simulink model "slcp"  (Simulink 6.3)
settings: Solver=ode5  SolverMode=SingleTasking  StartTime=0.0  StopTime=1000  FixedStep=.01  MaxStep=0.1  RelTol=1e-3  AbsTol=1e-6
PreLoadFcn:
  | initcp
undefined symbols (not defined in the file or in its folder): init_cond
libraries: fuzblock x1
CloseFcn:
  | AnimFigTitle = [winName, ': Cart & Pole Animation']; AnimFigH = findobj(0,'Name',AnimFigTitle); close(AnimFigH)
settings Model: Creator=pascal  LastModifiedBy=mhaselti  StrictBusMsg=None
settings DataIOCC: LimitDataPoints=off  SaveOutput=off  SaveTime=off
settings OptimizationCC: BlockReduction=off  BooleanDataType=off
settings DebuggingCC: SigSpecEnsureSampleTime=on  SolverPrmCheckMsg=none
settings HardwareCC: TargetUnknown=on
settings RTWCC: TemplateMakefile=grt_unix.tmf

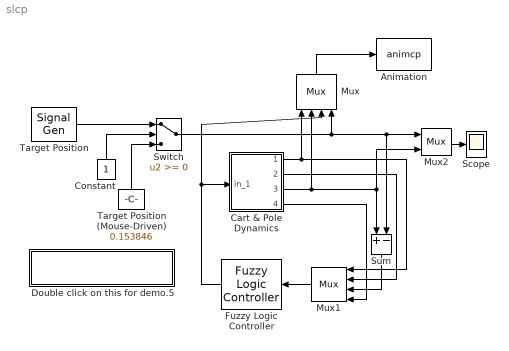
== system slcp ==
  Animation : S-Function  FunctionName=animcp
  Cart & Pole Dynamics : Subsystem  mask(Cart & Pole){init_cond =[0, 0, 0, 0],  specs =[1.0, 0.1, 1.0, 9.8]}
      mask prompts: init_cond  "Initial Conditions (angle, angular velocity, cart position and cart velocity):";  specs  "Physical Specifications (pole length, pole mass, cart mass and g):"
      mask help: Inverted Pendulum (cart & pole)
      mask init:
      | l=specs(1)/2;m=specs(2);mc=specs(3);g=specs(4);
      mask Help: Inverted Pendulum
      mask Display: plot(-4,-1,4,6,[0 3 2.8 -0.2 0],[1 5 5.15 1.15 1],[-1 -1 1 1 -1],[1 0 0 1 1],[-3.5 3.5],[0 0])
  Constant : Constant  Orientation=up
  Double click on this for demo.5 : Subsystem
      settings: OpenFcn=initcp
      mask Display: disp('Variable Initialization')
  Fuzzy Logic Controller : fuzblock/Fuzzy Logic  Controller  Orientation=left  fis=fismatrix
  Mux : Mux  Orientation=up
  Mux1 : Mux  Orientation=left
  Mux2 : Mux  Inputs=2
  Scope : Scope
      settings: TickLabels=on  TimeRange=10.000000  YMin=-2  YMax=2  DataFormat=Array
  Sum : Sum  Orientation=down  Inputs=+-  SaturateOnIntegerOverflow=on  InputSameDT=on
  Switch : Switch  SaturateOnIntegerOverflow=on  InputSameDT=on
  Target Position : SignalGenerator  WaveForm=square  Amplitude=1.500000  Frequency=0.628320  Units=rad/sec
  Target Position (Mouse-Driven) : Constant  Orientation=up  Value=0.153846
  wires:
  Target Position/1 -> Switch/1
  Constant/1 -> Switch/2
  Target Position (Mouse-Driven)/1 -> Switch/3
  Mux2/1 -> Scope/1
  Mux/1 -> Animation/1
  Cart & Pole Dynamics/4(out_4) -> Mux1/4
  Switch/1 -> Mux2/1, Sum/2, Mux/4
  Fuzzy Logic Controller/1 -> Mux/3, Cart & Pole Dynamics/1(in_1)
  Cart & Pole Dynamics/3(out_3) -> Mux2/2, Sum/1, Mux/2
  Cart & Pole Dynamics/1(out_1) -> Mux/1, Mux1/1
  Cart & Pole Dynamics/2(out_2) -> Mux1/2
  Sum/1 -> Mux1/3
  Mux1/1 -> Fuzzy Logic Controller/1

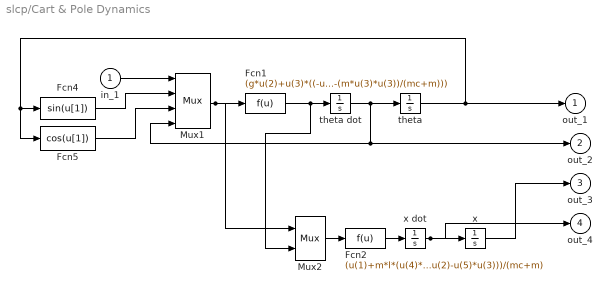
== system slcp/Cart & Pole Dynamics ==
  in_1 : Inport  Port=1  LatchInput=off  HoldInput=off
  Fcn1 : Fcn  Expr=(g*u(2)+u(3)*((-u(1)-m*l*u(4)*u(4)*u(2))/(mc+m)))/(l*(4/3-(m*u(3)*u(3))/(mc+m)))
  Fcn2 : Fcn  Expr=(u(1)+m*l*(u(4)*u(4)*u(2)-u(5)*u(3)))/(mc+m)
  Fcn4 : Fcn
  Fcn5 : Fcn  Expr=cos(u[1])
  Mux1 : Mux
  Mux2 : Mux  Inputs=[4,1]
  theta : Integrator  InitialCondition=init_cond(1)
  theta dot : Integrator  InitialCondition=init_cond(2)
  x : Integrator  InitialCondition=init_cond(3)
  x dot : Integrator  InitialCondition=init_cond(4)
  out_1 : Outport  InitialOutput=0
  out_2 : Outport  Port=2  InitialOutput=0
  out_3 : Outport  Port=3  InitialOutput=0
  out_4 : Outport  Port=4  InitialOutput=0
  wires:
  in_1/1 -> Mux1/1
  x/1 -> out_3/1
  x dot/1 -> out_4/1, x/1
  Mux1/1 -> Fcn1/1, Mux2/1
  Mux2/1 -> Fcn2/1
  Fcn2/1 -> x dot/1
  Fcn1/1 -> Mux2/2, theta dot/1
  theta dot/1 -> Mux1/4, out_2/1, theta/1
  Fcn4/1 -> Mux1/2
  Fcn5/1 -> Mux1/3
  theta/1 -> Fcn4/1, Fcn5/1, out_1/1

== system slcp/Double click on this for demo.5 ==
